simulink model "mracSimulink"  (R2017a)
settings: Solver=VariableStepAuto  StartTime=0.0  StopTime=50  RelTol=1e-3
settings Model: Creator=Herculano  LastModifiedBy=Herculano

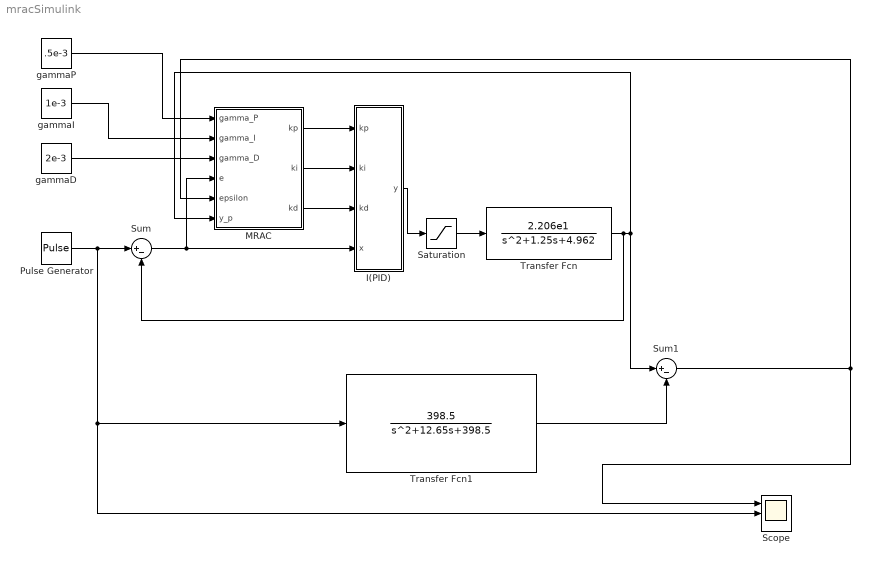
== system mracSimulink ==
  "I(PID) " : Subsystem
  MRAC : Subsystem
  Pulse Generator : DiscretePulseGenerator  PulseType=Time based  Amplitude=1e3  Period=3  PulseWidth=50  PhaseDelay=0.1
  Saturation : Saturate  UpperLimit=20000  LowerLimit=-20000
  Scope : Scope  NumInputPorts=3
  Sum : Sum  Inputs=|+-
  Sum1 : Sum  Inputs=|+-
  Transfer Fcn : TransferFcn  Numerator=[2.206e1]  Denominator=[1 1.25 4.962]
  Transfer Fcn1 : TransferFcn  Numerator=[398.5]  Denominator=[1 12.65 398.5]
  gammaD : Constant  Value=2e-3
  gammaI : Constant  Value=1e-3
  gammaP : Constant  Value=.5e-3
  wires:
  Pulse Generator/1 -> Transfer Fcn1/1, Scope/2, Sum/1
  Sum/1 -> "I(PID) "/4(x), MRAC/4("e ")
  Transfer Fcn1/1 -> Sum1/2
  Sum1/1 -> MRAC/5(epsilon), Scope/1
  Transfer Fcn/1 -> Sum/2, Sum1/1, MRAC/6(y_p)
  Saturation/1 -> Transfer Fcn/1
  "I(PID) "/1(y) -> Saturation/1
  gammaP/1 -> MRAC/1(gamma_P)
  gammaI/1 -> MRAC/2(gamma_I)
  gammaD/1 -> MRAC/3(gamma_D)
  MRAC/1(kp) -> "I(PID) "/1(kp)
  MRAC/2(ki) -> "I(PID) "/2(ki)
  MRAC/3(kd) -> "I(PID) "/3(kd)

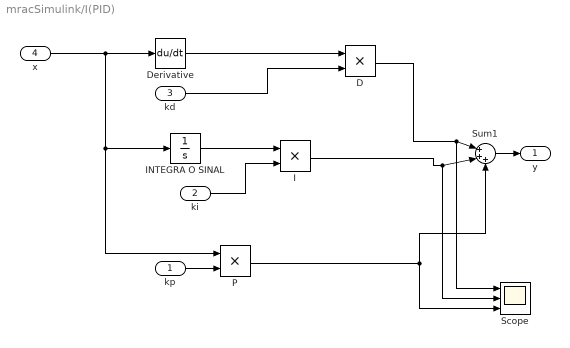
== system mracSimulink/I(PID)  ==
  kp : Inport
  ki : Inport  Port=2
  kd : Inport  Port=3
  x : Inport  Port=4
  D : Product
  Derivative : Derivative
  I : Product
  INTEGRA O SINAL : Integrator
  P : Product
  Scope : Scope  NumInputPorts=3
  Sum1 : Sum  Inputs=|+++
  y : Outport
  wires:
  Sum1/1 -> y/1
  I/1 -> Scope/2, Sum1/2
  INTEGRA O SINAL/1 -> I/1
  P/1 -> Sum1/3, Scope/3
  D/1 -> Scope/1, Sum1/1
  ki/1 -> I/2
  kp/1 -> P/2
  x/1 -> INTEGRA O SINAL/1, P/1, Derivative/1
  Derivative/1 -> D/1
  kd/1 -> D/2

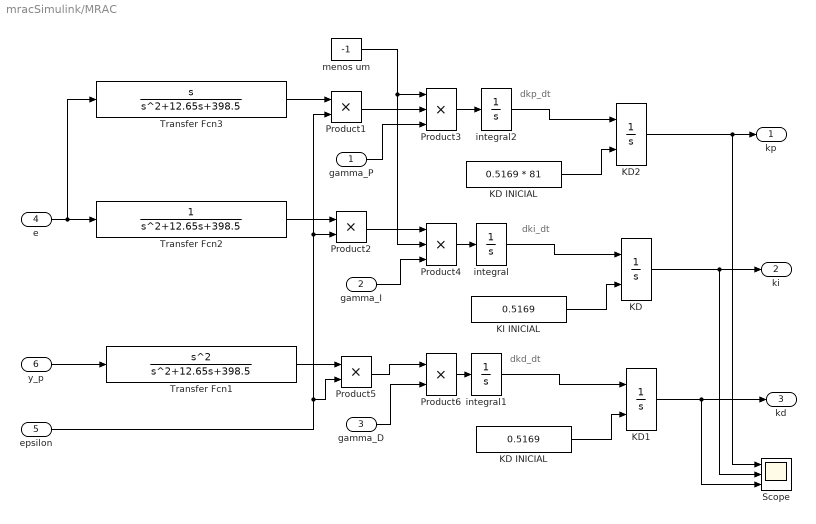
== system mracSimulink/MRAC ==
  note: dki_dt
  note: dkd_dt
  note: dkp_dt
  gamma_P : Inport
  gamma_I : Inport  Port=2
  gamma_D : Inport  Port=3
  "e " : Inport  Port=4
  epsilon : Inport  Port=5
  y_p : Inport  Port=6
  KD : Integrator  InitialConditionSource=external  InitialCondition=1000
  KD INICIAL : Constant  Value=0.5169
  "KD INICIAL " : Constant  Value=0.5169 * 81
  KD1 : Integrator  InitialConditionSource=external  InitialCondition=1000
  KD2 : Integrator  InitialConditionSource=external  InitialCondition=1000
  "KI INICIAL " : Constant  Value=0.5169
  Product{1..2,5..6} (4 alike) : Product
  Product3 : Product  Inputs=3
  Product4 : Product  Inputs=3
  Scope : Scope  NumInputPorts=3
  Transfer Fcn1 : TransferFcn  Numerator=[1 0 0]  Denominator=[1 12.65 398.5]
  Transfer Fcn2 : TransferFcn  Denominator=[1 12.65 398.5]
  Transfer Fcn3 : TransferFcn  Numerator=[1 0]  Denominator=[1 12.65 398.5]
  integral : Integrator
  integral1 : Integrator
  integral2 : Integrator
  menos um : Constant  Value=-1
  kp : Outport
  ki : Outport  Port=2
  kd : Outport  Port=3
  wires:
  "KI INICIAL "/1 -> KD/2
  KD/1 -> Scope/2, ki/1
  Transfer Fcn2/1 -> Product2/1
  Product2/1 -> Product4/1
  Product4/1 -> integral/1
  integral/1 -> KD/1
  gamma_D/1 -> Product6/2
  Transfer Fcn1/1 -> Product5/1
  epsilon/1 -> Product1/2, Product2/2, Product5/2
  y_p/1 -> Transfer Fcn1/1
  Product5/1 -> Product6/1
  Product6/1 -> integral1/1
  KD INICIAL/1 -> KD1/2
  integral1/1 -> KD1/1
  KD1/1 -> Scope/3, kd/1
  Transfer Fcn3/1 -> Product1/1
  "e "/1 -> Transfer Fcn3/1, Transfer Fcn2/1
  Product3/1 -> integral2/1
  "KD INICIAL "/1 -> KD2/2
  integral2/1 -> KD2/1
  KD2/1 -> Scope/1, kp/1
  menos um/1 -> Product3/1, Product4/2
  gamma_I/1 -> Product4/3
  gamma_P/1 -> Product3/3
  Product1/1 -> Product3/2
